simulink model "Ensamble_robot"  (R2016b)
settings: Solver=ode45  StartTime=0.0  StopTime=inf  RelTol=1e-3  EnableMultiTasking=on
undefined symbols (not defined in the file or in its folder): Brazo_1, Brazo_2, Ensamble_robot, Pinza, Pinza_1, RootPart, sigbuilder_block, Soporte, Torre
libraries: mblibv1 x28, simulink x12
settings Model: Creator=Alex3  LastModifiedBy=juan
settings DataIOCC: LimitDataPoints=on  SaveFormat=Array
settings OptimizationCC: LifeSpan=inf
settings DebuggingCC: SFUnexpectedBacktrackingDiag=warning  SFNoUnconditionalDefaultTransitionDiag=warning  SFExecutionAtInitializationDiag=none
settings HardwareCC: ProdBitPerPointer=32  ProdBitPerSizeT=32  ProdBitPerPtrDiffT=32  ProdLargestAtomicFloat=None  ProdIntDivRoundTo=Undefined  ProdEndianess=Unspecified  ProdWordSize=32  ProdHWDeviceType=32-bit Generic
settings ModelReferenceCC: PropagateSignalLabelsOutOfModel=off
settings GRTTargetCC: TargetLangStandard=C89/C90 (ANSI)  GeneratePreprocessorConditionals=Disable all
settings ConfigComp: CovMetricSettings=dw  CovHtmlReporting=on  CovSaveCumulativeToWorkspaceVar=on  CovSaveSingleToWorkspaceVar=on  CovExternalEMLEnable=off
settings SimMechanicsCC: VisOnUpdateDiagram=on  VisDuringSimulation=on
settings ConfigurationSet: Description=SimMechanics 2G

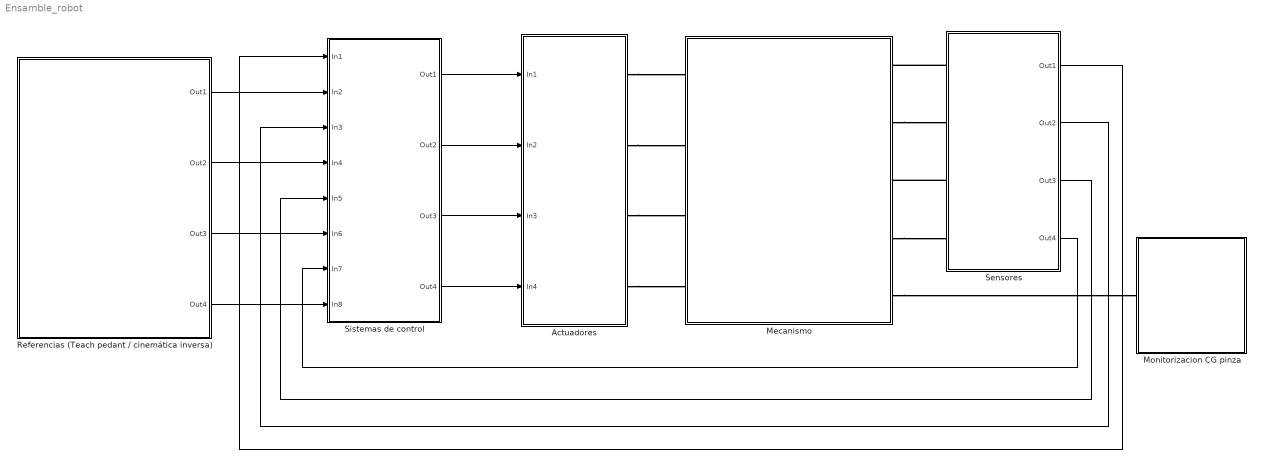
== system Ensamble_robot ==
  Actuadores : Subsystem
      mask Display: image('masks/motor.jpg');
  Mecanismo : Subsystem
      mask Display: image('masks/mascara_robot.png');
  "Monitorizacion CG pinza " : Subsystem
      mask Display: image('masks/orion_console_2_sm.jpg');
  Referencias (Teach pedant / cinemática inversa) : Subsystem
      mask Display: image('masks/_TEACHPD.GIF');
  Sensores : Subsystem
      mask Display: image('masks/encoders4.png');
  Sistemas de control : Subsystem
      mask Display: image('masks/pids4.png');
  wires:
  Sensores/1(Out1) -> Sistemas de control/1(In1)
  Sensores/2(Out2) -> Sistemas de control/3(In3)
  Sensores/3(Out3) -> Sistemas de control/5(In5)
  Sensores/4(Out4) -> Sistemas de control/7(In7)
  Sistemas de control/1(Out1) -> Actuadores/1(In1)
  Sistemas de control/2(Out2) -> Actuadores/2(In2)
  Sistemas de control/3(Out3) -> Actuadores/3(In3)
  Sistemas de control/4(Out4) -> Actuadores/4(In4)
  Referencias (Teach pedant / cinemática inversa)/1(Out1) -> Sistemas de control/2(In2)
  Referencias (Teach pedant / cinemática inversa)/2(Out2) -> Sistemas de control/4(In4)
  Referencias (Teach pedant / cinemática inversa)/3(Out3) -> Sistemas de control/6(In6)
  Referencias (Teach pedant / cinemática inversa)/4(Out4) -> Sistemas de control/8(In8)
  connections:
  Mecanismo/RConn5 -- "Monitorizacion CG pinza "/LConn1
  Actuadores/RConn1 -- Mecanismo/LConn1
  Actuadores/RConn2 -- Mecanismo/LConn2
  Actuadores/RConn3 -- Mecanismo/LConn3
  Actuadores/RConn4 -- Mecanismo/LConn4
  Sensores/LConn1 -- Mecanismo/RConn1
  Mecanismo/RConn2 -- Sensores/LConn2
  Sensores/LConn3 -- Mecanismo/RConn3
  Mecanismo/RConn4 -- Sensores/LConn4

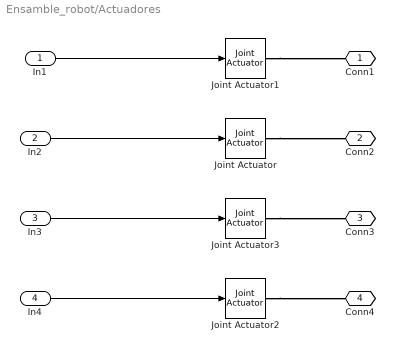
== system Ensamble_robot/Actuadores ==
  In1 : Inport
  In2 : Inport  Port=2
  In3 : Inport  Port=3
  In4 : Inport  Port=4
  Joint Actuator : mblibv1/Sensors &  Actuators/Joint Actuator  UpdateFromCAD=off  PhysicalDomain=Mechanical  PortType=blob  ActuationStyle=Motion  AngleUnits=deg  ArcVelocityUnits=deg/s  ArcAccelerationUnits=deg/s^2  CoordPositionUnits=mm  VelocityUnits=mm/s  AccelerationUnits=mm/s^2  ForceUnits=N  TorqueUnits=N*m  ActiveIO=on  Width=3  DialogClass=MechanicalActuatorBlock  Primitive=P1  ReferenceFrame=Absolute (World)
  Joint Actuator1 : mblibv1/Sensors &  Actuators/Joint Actuator  UpdateFromCAD=off  PhysicalDomain=Mechanical  PortType=blob  ActuationStyle=Motion  AngleUnits=rad  ArcVelocityUnits=rad/s  ArcAccelerationUnits=rad/s^2  CoordPositionUnits=mm  VelocityUnits=mm/s  AccelerationUnits=mm/s^2  ForceUnits=N  TorqueUnits=N*m  ActiveIO=on  Width=3  DialogClass=MechanicalActuatorBlock  Primitive=R1  ReferenceFrame=Absolute (World)
  Joint Actuator2 : mblibv1/Sensors &  Actuators/Joint Actuator  UpdateFromCAD=off  PhysicalDomain=Mechanical  PortType=blob  ActuationStyle=Motion  AngleUnits=rad  ArcVelocityUnits=rad/s  ArcAccelerationUnits=rad/s^2  CoordPositionUnits=mm  VelocityUnits=mm/s  AccelerationUnits=mm/s^2  ForceUnits=N  TorqueUnits=N*m  ActiveIO=on  Width=3  DialogClass=MechanicalActuatorBlock  Primitive=R1  ReferenceFrame=Absolute (World)
  Joint Actuator3 : mblibv1/Sensors &  Actuators/Joint Actuator  UpdateFromCAD=off  PhysicalDomain=Mechanical  PortType=blob  ActuationStyle=Motion  AngleUnits=rad  ArcVelocityUnits=rad/s  ArcAccelerationUnits=rad/s^2  CoordPositionUnits=mm  VelocityUnits=mm/s  AccelerationUnits=mm/s^2  ForceUnits=N  TorqueUnits=N*m  ActiveIO=on  Width=3  DialogClass=MechanicalActuatorBlock  Primitive=R1  ReferenceFrame=Absolute (World)
  Conn1 : PMIOPort  Port=1  Side=Right
  Conn2 : PMIOPort  Port=2  Side=Right
  Conn3 : PMIOPort  Port=3  Side=Right
  Conn4 : PMIOPort  Port=4  Side=Right
  wires:
  In1/1 -> Joint Actuator1/1
  In4/1 -> Joint Actuator2/1
  In3/1 -> Joint Actuator3/1
  In2/1 -> Joint Actuator/1
  connections:
  Joint Actuator2/RConn1 -- Conn4/RConn1
  Joint Actuator1/RConn1 -- Conn1/RConn1
  Joint Actuator3/RConn1 -- Conn3/RConn1
  Joint Actuator/RConn1 -- Conn2/RConn1

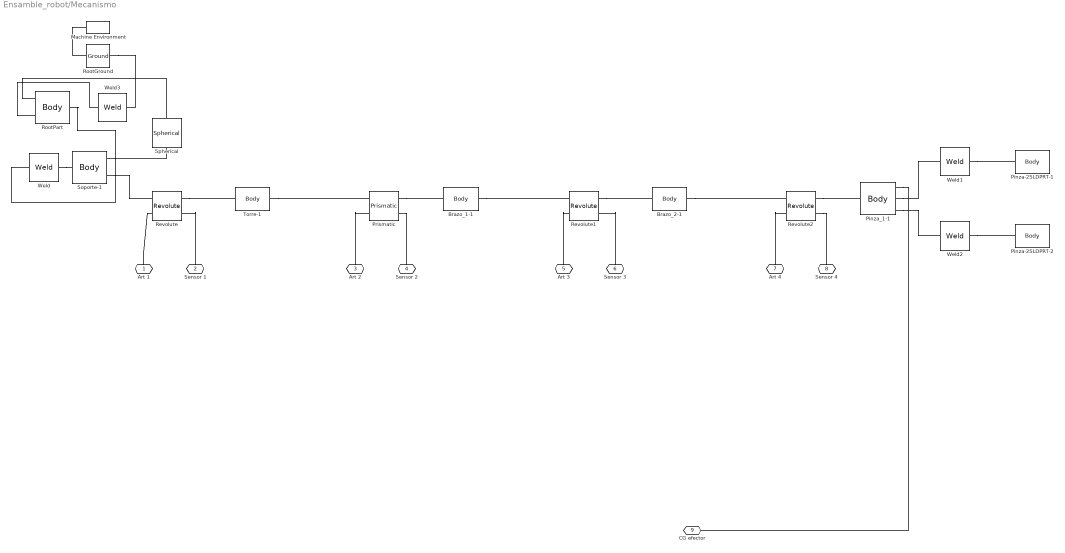
== system Ensamble_robot/Mecanismo ==
  Brazo_1-1 : mblibv1/Bodies/Body  LConnTagsString=CS2  RConnTagsString=CS3  UpdateFromCAD=on  PMImportedID=Brazo_1-1  DialogClass=MechanicalBodyBlock  Mass=5.04274  MassUnits=kg  InertiaUnits=kg*m^2  Inertia=[0.0173518,0.0122763,1.33704e-09;0.0122763,0.106444,-1.19326e-09;1.33704e-09,-1.19326e-09,0.102671]  Shape=Cylinder  ShapeDims=[1 1]  ShapeUnits=m  ShapeUse=false  Density=1  DensityUnits=kg/m^3  DensityUse=false  GraphicsMode=GFXFILE  GraphicsFileName=Ensamble_robot - Brazo_1-1.STL  BodyColorSelMode=COLORPALETTE  BodyColor=[1;1;1]  AttachedToCS=CS1  CG=Right$CG$[0.204832 0.0464629 2.69197e-09]$WORLD$WORLD$m$[1 0 0;0 1 0;0 0 1]$3x3 Transform$rad$WORLD$false$Brazo_1-1::CG(AUTOGEN)  WorkingFrames=Right$CS1$[0.45 0.0499751 0]$WORLD$WORLD$m$[1 0 0;0 1 0;0 0 1]$3x3 Transform$rad$WORLD$false$Brazo_1-1::CS1(AUTOGEN)#Left$CS2$[0 0.149975 0.045]$WORLD$WORLD$m$[1 0 0;0 1 0;0 0 1]$3x3 Transform$rad$WORLD$true$Brazo_1-1:-:Torre-1::Brazo_1-1(AUTOGEN)#Right$CS3$[0.45 0.0299751 0]$WORLD$WORLD$m$[1 0 0;0 1 0;0 0 1]$3x3 Transform$rad$WORLD$true$Brazo_1-1:-:Brazo_2-1::Brazo_1-1(AUTOGEN)  CGPos=[0.204832 0.0464629 2.69197e-09]  CGRot=[1 0 0;0 1 0;0 0 1]  CS0Pos=[]  CS0Rot=[]  CS1Pos=[0.45 0.0499751 0]  CS1Rot=[1 0 0;0 1 0;0 0 1]  CS2Pos=[0 0.149975 0.045]  CS2Rot=[1 0 0;0 1 0;0 0 1]  CS3Pos=[0.45 0.0299751 0]  CS3Rot=[1 0 0;0 1 0;0 0 1]  CS4Pos=[]  CS4Rot=[]  CS5Pos=[]  CS5Rot=[]  CS6Pos=[]  CS6Rot=[]  CS7Pos=[]  CS7Rot=[]  CS8Pos=[]  CS8Rot=[]  CS9Pos=[]  CS9Rot=[]  CS10Pos=[]  CS10Rot=[]  CS11Pos=[]  CS11Rot=[]  CS12Pos=[]  CS12Rot=[]  CS13Pos=[]  CS13Rot=[]  CS14Pos=[]  CS14Rot=[]  CS15Pos=[]  CS15Rot=[]  CS16Pos=[]  CS16Rot=[]  CS17Pos=[]  CS17Rot=[]  CS18Pos=[]  CS18Rot=[]  CS19Pos=[]  CS19Rot=[]  CS20Pos=[]  CS20Rot=[]
  Brazo_2-1 : mblibv1/Bodies/Body  LConnTagsString=CS2  RConnTagsString=CS3  UpdateFromCAD=on  PMImportedID=Brazo_2-1  DialogClass=MechanicalBodyBlock  Mass=1.88667  MassUnits=kg  InertiaUnits=kg*m^2  Inertia=[0.00269492,0.000426403,-1.18231e-09;0.000426403,0.0126019,2.20098e-09;-1.18231e-09,2.20098e-09,0.0117797]  Shape=Cylinder  ShapeDims=[1 1]  ShapeUnits=m  ShapeUse=false  Density=1  DensityUnits=kg/m^3  DensityUse=false  GraphicsMode=GFXFILE  GraphicsFileName=Ensamble_robot - Brazo_2-1.STL  BodyColorSelMode=COLORPALETTE  BodyColor=[1;1;1]  AttachedToCS=CS1  CG=Right$CG$[0.507024 -0.0192513 -1.13579e-08]$WORLD$WORLD$m$[1 0 0;0 1 0;0 0 1]$3x3 Transform$rad$WORLD$false$Brazo_2-1::CG(AUTOGEN)  WorkingFrames=Right$CS1$[0.45 -0.0500249 0]$WORLD$WORLD$m$[1 0 0;0 1 0;0 0 1]$3x3 Transform$rad$WORLD$false$Brazo_2-1::CS1(AUTOGEN)#Left$CS2$[0.45 0.0299751 0]$WORLD$WORLD$m$[1 0 0;0 1 0;0 0 1]$3x3 Transform$rad$WORLD$true$Brazo_1-1:-:Brazo_2-1::Brazo_2-1(AUTOGEN)#Right$CS3$[0.65 -0.0200249 0]$WORLD$WORLD$m$[1 0 0;0 1 0;0 0 1]$3x3 Transform$rad$WORLD$true$Brazo_2-1:-:Pinza_1-1::Brazo_2-1(AUTOGEN)  CGPos=[0.507024 -0.0192513 -1.13579e-08]  CGRot=[1 0 0;0 1 0;0 0 1]  CS0Pos=[]  CS0Rot=[]  CS1Pos=[0.45 -0.0500249 0]  CS1Rot=[1 0 0;0 1 0;0 0 1]  CS2Pos=[0.45 0.0299751 0]  CS2Rot=[1 0 0;0 1 0;0 0 1]  CS3Pos=[0.65 -0.0200249 0]  CS3Rot=[1 0 0;0 1 0;0 0 1]  CS4Pos=[]  CS4Rot=[]  CS5Pos=[]  CS5Rot=[]  CS6Pos=[]  CS6Rot=[]  CS7Pos=[]  CS7Rot=[]  CS8Pos=[]  CS8Rot=[]  CS9Pos=[]  CS9Rot=[]  CS10Pos=[]  CS10Rot=[]  CS11Pos=[]  CS11Rot=[]  CS12Pos=[]  CS12Rot=[]  CS13Pos=[]  CS13Rot=[]  CS14Pos=[]  CS14Rot=[]  CS15Pos=[]  CS15Rot=[]  CS16Pos=[]  CS16Rot=[]  CS17Pos=[]  CS17Rot=[]  CS18Pos=[]  CS18Rot=[]  CS19Pos=[]  CS19Rot=[]  CS20Pos=[]  CS20Rot=[]
  Machine Environment : mblibv1/Bodies/Machine Environment  PortType=env  PhysicalDomain=Mechanical  DialogTemplateClass=MECH.MachineEnvironment  SyncWhenCopied=off  Gravity=[0 -9.81 0]  GravityUnits=m/s^2  GravityAsSignal=off  Dimensionality=Auto-detect  AnalysisType=Forward dynamics  LinearAssemblyTolerance=1e-3  LinearAssemblyToleranceUnits=m  AngularAssemblyTolerance=1e-3  AngularAssemblyToleranceUnits=rad  ConstraintSolverType=Stabilizing  ConstraintRelTolerance=1e-4  ConstraintAbsTolerance=1e-4  UseRobustSingularityHandling=off  RedundancyAnalysisToleranceType=Automatically select tolerance  RedundancyAnalysisTolerance=1e-14  StatePerturbationType=Fixed  PerturbationSize=1e-5  VisualizeMachine=on  BodyVisualizationType=Use model default body geometries  BodyColorSelMode=Use model default  DefaultBodyColor=[1 0 0]
  Pinza-2SLDPRT-1 : mblibv1/Bodies/Body  LConnTagsString=CS2  UpdateFromCAD=on  PMImportedID=Pinza-2SLDPRT-1  DialogClass=MechanicalBodyBlock  Mass=0.01755  MassUnits=kg  InertiaUnits=kg*m^2  Inertia=[5.56763e-07,0,0;0,7.2684e-06,0;0,0,6.78476e-06]  Shape=Cylinder  ShapeDims=[1 1]  ShapeUnits=m  ShapeUse=false  Density=1  DensityUnits=kg/m^3  DensityUse=false  GraphicsMode=GFXFILE  GraphicsFileName=Ensamble_robot - Pinza-2SLDPRT-1.STL  BodyColorSelMode=COLORPALETTE  BodyColor=[0.894118;0.913725;0.929412]  AttachedToCS=CS1  CG=Right$CG$[0.705013 -0.0950249 -0.0525]$WORLD$WORLD$m$[1 0 0;0 0 1;0 -1 0]$3x3 Transform$rad$WORLD$false$Pinza-2SLDPRT-1::CG(AUTOGEN)  WorkingFrames=Right$CS1$[0.697 -0.0950249 -0.05]$WORLD$WORLD$m$[1 0 0;0 0 1;0 -1 0]$3x3 Transform$rad$WORLD$false$Pinza-2SLDPRT-1::CS1(AUTOGEN)#Left$CS2$[0.672 -0.105025 -0.055]$WORLD$WORLD$m$[1 0 0;0 1 0;0 0 1]$3x3 Transform$rad$WORLD$true$Pinza-2SLDPRT-1:-:Pinza_1-1::Pinza-2SLDPRT-1(AUTOGEN)  CGPos=[0.705013 -0.0950249 -0.0525]  CGRot=[1 0 0;0 0 1;0 -1 0]  CS0Pos=[]  CS0Rot=[]  CS1Pos=[0.697 -0.0950249 -0.05]  CS1Rot=[1 0 0;0 0 1;0 -1 0]  CS2Pos=[0.672 -0.105025 -0.055]  CS2Rot=[1 0 0;0 1 0;0 0 1]  CS3Pos=[]  CS3Rot=[]  CS4Pos=[]  CS4Rot=[]  CS5Pos=[]  CS5Rot=[]  CS6Pos=[]  CS6Rot=[]  CS7Pos=[]  CS7Rot=[]  CS8Pos=[]  CS8Rot=[]  CS9Pos=[]  CS9Rot=[]  CS10Pos=[]  CS10Rot=[]  CS11Pos=[]  CS11Rot=[]  CS12Pos=[]  CS12Rot=[]  CS13Pos=[]  CS13Rot=[]  CS14Pos=[]  CS14Rot=[]  CS15Pos=[]  CS15Rot=[]  CS16Pos=[]  CS16Rot=[]  CS17Pos=[]  CS17Rot=[]  CS18Pos=[]  CS18Rot=[]  CS19Pos=[]  CS19Rot=[]  CS20Pos=[]  CS20Rot=[]
  Pinza-2SLDPRT-2 : mblibv1/Bodies/Body  LConnTagsString=CS2  UpdateFromCAD=on  PMImportedID=Pinza-2SLDPRT-2  DialogClass=MechanicalBodyBlock  Mass=0.01755  MassUnits=kg  InertiaUnits=kg*m^2  Inertia=[5.56763e-07,0,0;0,7.2684e-06,0;0,0,6.78476e-06]  Shape=Cylinder  ShapeDims=[1 1]  ShapeUnits=m  ShapeUse=false  Density=1  DensityUnits=kg/m^3  DensityUse=false  GraphicsMode=GFXFILE  GraphicsFileName=Ensamble_robot - Pinza-2SLDPRT-2.STL  BodyColorSelMode=COLORPALETTE  BodyColor=[0.894118;0.913725;0.929412]  AttachedToCS=CS1  CG=Right$CG$[0.705013 -0.0950249 0.0525]$WORLD$WORLD$m$[1 0 0;0 0 -1;0 1 0]$3x3 Transform$rad$WORLD$false$Pinza-2SLDPRT-2::CG(AUTOGEN)  WorkingFrames=Right$CS1$[0.697 -0.0950249 0.05]$WORLD$WORLD$m$[1 0 0;0 0 -1;0 1 0]$3x3 Transform$rad$WORLD$false$Pinza-2SLDPRT-2::CS1(AUTOGEN)#Left$CS2$[0.672 -0.105025 0.055]$WORLD$WORLD$m$[1 0 0;0 1 0;0 0 1]$3x3 Transform$rad$WORLD$true$Pinza-2SLDPRT-2:-:Pinza_1-1::Pinza-2SLDPRT-2(AUTOGEN)  CGPos=[0.705013 -0.0950249 0.0525]  CGRot=[1 0 0;0 0 -1;0 1 0]  CS0Pos=[]  CS0Rot=[]  CS1Pos=[0.697 -0.0950249 0.05]  CS1Rot=[1 0 0;0 0 -1;0 1 0]  CS2Pos=[0.672 -0.105025 0.055]  CS2Rot=[1 0 0;0 1 0;0 0 1]  CS3Pos=[]  CS3Rot=[]  CS4Pos=[]  CS4Rot=[]  CS5Pos=[]  CS5Rot=[]  CS6Pos=[]  CS6Rot=[]  CS7Pos=[]  CS7Rot=[]  CS8Pos=[]  CS8Rot=[]  CS9Pos=[]  CS9Rot=[]  CS10Pos=[]  CS10Rot=[]  CS11Pos=[]  CS11Rot=[]  CS12Pos=[]  CS12Rot=[]  CS13Pos=[]  CS13Rot=[]  CS14Pos=[]  CS14Rot=[]  CS15Pos=[]  CS15Rot=[]  CS16Pos=[]  CS16Rot=[]  CS17Pos=[]  CS17Rot=[]  CS18Pos=[]  CS18Rot=[]  CS19Pos=[]  CS19Rot=[]  CS20Pos=[]  CS20Rot=[]
  Pinza_1-1 : mblibv1/Bodies/Body  LConnTagsString=CS2  RConnTagsString=CG|CS3|CS4  UpdateFromCAD=on  PMImportedID=Pinza_1-1  DialogClass=MechanicalBodyBlock  Mass=1.1552  MassUnits=kg  InertiaUnits=kg*m^2  Inertia=[0.00139548,9.82419e-05,0;9.82419e-05,0.00107204,0;0,0,0.00130274]  Shape=Cylinder  ShapeDims=[1 1]  ShapeUnits=m  ShapeUse=false  Density=1  DensityUnits=kg/m^3  DensityUse=false  GraphicsMode=GFXFILE  GraphicsFileName=Ensamble_robot - Pinza_1-1.STL  BodyColorSelMode=COLORPALETTE  BodyColor=[0.89412 0.91373 0.92941]  AttachedToCS=CS1  CG=Right$CG$[0.653502 -0.0707388 0]$WORLD$WORLD$m$[1 0 0;0 1 0;0 0 1]$3x3 Transform$rad$WORLD$true$Pinza_1-1::CG(AUTOGEN)  WorkingFrames=Right$CS1$[0.65 -0.110025 0]$WORLD$WORLD$m$[1 0 0;0 1 0;0 0 1]$3x3 Transform$rad$WORLD$false$Pinza_1-1::CS1(AUTOGEN)#Left$CS2$[0.65 -0.0200249 0]$WORLD$WORLD$m$[1 0 0;0 1 0;0 0 1]$3x3 Transform$rad$WORLD$true$Brazo_2-1:-:Pinza_1-1::Pinza_1-1(AUTOGEN)#Right$CS3$[0.672 -0.105025 -0.055]$WORLD$WORLD$m$[1 0 0;0 1 0;0 0 1]$3x3 Transform$rad$WORLD$true$Pinza-2SLDPRT-1:-:Pinza_1-1::Pinza_1-1(AUTOGEN)#Right$CS4$[0.672 -0.105025 0.055]$WORLD$WORLD$m$[1 0 0;0 1 0;0 0 1]$3x3 Transform$rad$WORLD$true$Pinza-2SLDPRT-2:-:Pinza_1-1::Pinza_1-1(AUTOGEN)  CGPos=[0.653502 -0.0707388 0]  CGRot=[1 0 0;0 1 0;0 0 1]  CS0Pos=[]  CS0Rot=[]  CS1Pos=[0.65 -0.110025 0]  CS1Rot=[1 0 0;0 1 0;0 0 1]  CS2Pos=[0.65 -0.0200249 0]  CS2Rot=[1 0 0;0 1 0;0 0 1]  CS3Pos=[0.672 -0.105025 -0.055]  CS3Rot=[1 0 0;0 1 0;0 0 1]  CS4Pos=[0.672 -0.105025 0.055]  CS4Rot=[1 0 0;0 1 0;0 0 1]  CS5Pos=[]  CS5Rot=[]  CS6Pos=[]  CS6Rot=[]  CS7Pos=[]  CS7Rot=[]  CS8Pos=[]  CS8Rot=[]  CS9Pos=[]  CS9Rot=[]  CS10Pos=[]  CS10Rot=[]  CS11Pos=[]  CS11Rot=[]  CS12Pos=[]  CS12Rot=[]  CS13Pos=[]  CS13Rot=[]  CS14Pos=[]  CS14Rot=[]  CS15Pos=[]  CS15Rot=[]  CS16Pos=[]  CS16Rot=[]  CS17Pos=[]  CS17Rot=[]  CS18Pos=[]  CS18Rot=[]  CS19Pos=[]  CS19Rot=[]  CS20Pos=[]  CS20Rot=[]
  Prismatic : mblibv1/Joints/Prismatic  LConnTagsString=__newl0|SA1  RConnTagsString=__newr0|SA1  UpdateFromCAD=on  PMImportedID=Brazo_1-1:-:Torre-1  NumSAPorts=2  CutJoint=off  MarkAsCut=off  Primitives=prismatic  PrimitiveProps=P1$World$[0,-1,0]$prismatic  DialogClass=JointBlock  P1Axis=[0,-1,0]
  Revolute : mblibv1/Joints/Revolute  LConnTagsString=__newl0|SA1  RConnTagsString=__newr0|SA1  UpdateFromCAD=on  PMImportedID=Soporte-1:-:Torre-1  NumSAPorts=2  CutJoint=off  MarkAsCut=off  Primitives=prismatic  PrimitiveProps=R1$World$[0,-1,0]$revolute  DialogClass=JointBlock  R1Axis=[0,-1,0]
  Revolute1 : mblibv1/Joints/Revolute  LConnTagsString=__newl0|SA1  RConnTagsString=__newr0|SA1  UpdateFromCAD=on  PMImportedID=Brazo_1-1:-:Brazo_2-1  NumSAPorts=2  CutJoint=off  MarkAsCut=off  Primitives=prismatic  PrimitiveProps=R1$World$[0,-1,0]$revolute  DialogClass=JointBlock  R1Axis=[0,-1,0]
  Revolute2 : mblibv1/Joints/Revolute  LConnTagsString=__newl0|SA1  RConnTagsString=__newr0|SA1  UpdateFromCAD=on  PMImportedID=Brazo_2-1:-:Pinza_1-1  NumSAPorts=2  CutJoint=off  MarkAsCut=off  Primitives=prismatic  PrimitiveProps=R1$World$[0,-1,0]$revolute  DialogClass=JointBlock  R1Axis=[0,-1,0]
  RootGround : mblibv1/Bodies/Ground  UpdateFromCAD=on  PMImportedID=RootGround  LeftPortType=env  RightPortType=workingframe  PhysicalDomain=Mechanical  DialogClass=GroundBlock  CoordPosition=[0.0659419,0.00229338,1.11665e-06]  CoordPositionUnits=m  StateVectorMgrId=-1  MachineId=[0 0]  ShowEnvPort=on  ParameterChecksum=[1902267943, 726416014, 765096310, 2272254341]  TopologyChecksum=[1063915244, 2503524642, 3963338569, 4138555748]
  RootPart : mblibv1/Bodies/Body  LConnTagsString=CS3|CS4  RConnTagsString=CS2  UpdateFromCAD=on  PMImportedID=Ensamble_robot/RootPart  DialogClass=MechanicalBodyBlock  Mass=0  MassUnits=kg  InertiaUnits=kg*m^2  Inertia=[0,0,0;0,0,0;0,0,0]  Shape=Cylinder  ShapeDims=[1 1]  ShapeUnits=m  ShapeUse=false  Density=1  DensityUnits=kg/m^3  DensityUse=false  GraphicsMode=MACHINE_DEFAULT  BodyColorSelMode=MACHINE_DEFAULT  BodyColor=[1;0;0]  AttachedToCS=CS1  CG=Right$CG$[0.0659419 0.00229338 1.11665e-06]$WORLD$WORLD$m$[1 0 0;0 1 0;0 0 1]$3x3 Transform$rad$WORLD$false$Ensamble_robot/RootPart::CG(AUTOGEN)  WorkingFrames=Right$CS1$[0 0 0]$WORLD$WORLD$m$[1 0 0;0 1 0;0 0 1]$3x3 Transform$rad$WORLD$false$Ensamble_robot/RootPart::CS1(AUTOGEN)#Right$CS2$[-0.119346 -0.242891 4.53911e-06]$WORLD$WORLD$m$[1 0 0;0 1 0;0 0 1]$3x3 Transform$rad$WORLD$true$Ensamble_robot/RootPart:-:Soporte-1::Ensamble_robot/RootPart(AUTOGEN)#Left$CS3$[0 0 0]$WORLD$WORLD$m$[1 0 0;0 1 0;0 0 1]$3x3 Transform$rad$WORLD$true$:-:Ensamble_robot/RootPart::Ensamble_robot/RootPart(AUTOGEN)#Left$CS4$[0.0659419 0.00229338 1.11665e-06]$WORLD$WORLD$m$[1 0 0;0 1 0;0 0 1]$3x3 Transform$rad$WORLD$true$Ensamble_robot/RootPart:-:RootGround::Ensamble_robot/RootPart(AUTOGEN)  CGPos=[0.0659419 0.00229338 1.11665e-06]  CGRot=[1 0 0;0 1 0;0 0 1]  CS0Pos=[]  CS0Rot=[]  CS1Pos=[0 0 0]  CS1Rot=[1 0 0;0 1 0;0 0 1]  CS2Pos=[-0.119346 -0.242891 4.53911e-06]  CS2Rot=[1 0 0;0 1 0;0 0 1]  CS3Pos=[0 0 0]  CS3Rot=[1 0 0;0 1 0;0 0 1]  CS4Pos=[0.0659419 0.00229338 1.11665e-06]  CS4Rot=[1 0 0;0 1 0;0 0 1]  CS5Pos=[]  CS5Rot=[]  CS6Pos=[]  CS6Rot=[]  CS7Pos=[]  CS7Rot=[]  CS8Pos=[]  CS8Rot=[]  CS9Pos=[]  CS9Rot=[]  CS10Pos=[]  CS10Rot=[]  CS11Pos=[]  CS11Rot=[]  CS12Pos=[]  CS12Rot=[]  CS13Pos=[]  CS13Rot=[]  CS14Pos=[]  CS14Rot=[]  CS15Pos=[]  CS15Rot=[]  CS16Pos=[]  CS16Rot=[]  CS17Pos=[]  CS17Rot=[]  CS18Pos=[]  CS18Rot=[]  CS19Pos=[]  CS19Rot=[]  CS20Pos=[]  CS20Rot=[]
  Soporte-1 : mblibv1/Bodies/Body  LConnTagsString=CS2  RConnTagsString=CS3|CS4  UpdateFromCAD=on  PMImportedID=Soporte-1  DialogClass=MechanicalBodyBlock  Mass=6.83887  MassUnits=kg  InertiaUnits=kg*m^2  Inertia=[0.0271292,0.00214532,-1.0763e-06;0.00214532,0.102791,-1.48243e-06;-1.0763e-06,-1.48243e-06,0.0878129]  Shape=Cylinder  ShapeDims=[1 1]  ShapeUnits=m  ShapeUse=false  Density=1  DensityUnits=kg/m^3  DensityUse=false  GraphicsMode=GFXFILE  GraphicsFileName=Ensamble_robot - Soporte-1.STL  BodyColorSelMode=COLORPALETTE  BodyColor=[1;1;1]  AttachedToCS=CS1  CG=Right$CG$[-0.119346 -0.242891 4.53911e-06]$WORLD$WORLD$m$[1 0 0;0 1 0;0 0 1]$3x3 Transform$rad$WORLD$false$Soporte-1::CG(AUTOGEN)  WorkingFrames=Right$CS1$[0 -0.29 0]$WORLD$WORLD$m$[1 0 0;0 1 0;0 0 1]$3x3 Transform$rad$WORLD$false$Soporte-1::CS1(AUTOGEN)#Left$CS2$[-0.119346 -0.242891 4.53911e-06]$WORLD$WORLD$m$[1 0 0;0 1 0;0 0 1]$3x3 Transform$rad$WORLD$true$Ensamble_robot/RootPart:-:Soporte-1::Soporte-1(AUTOGEN)#Right$CS3$[0 0 0]$WORLD$WORLD$m$[1 0 0;0 1 0;0 0 1]$3x3 Transform$rad$WORLD$true$:-:Ensamble_robot/RootPart::Soporte-1(AUTOGEN)#Right$CS4$[0 -0.23 0]$WORLD$WORLD$m$[1 0 0;0 1 0;0 0 1]$3x3 Transform$rad$WORLD$true$Soporte-1:-:Torre-1::Soporte-1(AUTOGEN)  CGPos=[-0.119346 -0.242891 4.53911e-06]  CGRot=[1 0 0;0 1 0;0 0 1]  CS0Pos=[]  CS0Rot=[]  CS1Pos=[0 -0.29 0]  CS1Rot=[1 0 0;0 1 0;0 0 1]  CS2Pos=[-0.119346 -0.242891 4.53911e-06]  CS2Rot=[1 0 0;0 1 0;0 0 1]  CS3Pos=[0 0 0]  CS3Rot=[1 0 0;0 1 0;0 0 1]  CS4Pos=[0 -0.23 0]  CS4Rot=[1 0 0;0 1 0;0 0 1]  CS5Pos=[]  CS5Rot=[]  CS6Pos=[]  CS6Rot=[]  CS7Pos=[]  CS7Rot=[]  CS8Pos=[]  CS8Rot=[]  CS9Pos=[]  CS9Rot=[]  CS10Pos=[]  CS10Rot=[]  CS11Pos=[]  CS11Rot=[]  CS12Pos=[]  CS12Rot=[]  CS13Pos=[]  CS13Rot=[]  CS14Pos=[]  CS14Rot=[]  CS15Pos=[]  CS15Rot=[]  CS16Pos=[]  CS16Rot=[]  CS17Pos=[]  CS17Rot=[]  CS18Pos=[]  CS18Rot=[]  CS19Pos=[]  CS19Rot=[]  CS20Pos=[]  CS20Rot=[]
  Spherical : mblibv1/Joints/Spherical  LConnTagsString=__newl0  RConnTagsString=__newr0  UpdateFromCAD=on  PMImportedID=:-:Ensamble_robot/RootPart  NumSAPorts=0  CutJoint=off  MarkAsCut=off  Primitives=spherical  PrimitiveProps=S$WORLD$[0,0,0]$spherical  DialogClass=JointBlock  SAxis=[0,0,0]
  Torre-1 : mblibv1/Bodies/Body  LConnTagsString=CS2  RConnTagsString=CS3  UpdateFromCAD=on  PMImportedID=Torre-1  DialogClass=MechanicalBodyBlock  Mass=12.906  MassUnits=kg  InertiaUnits=kg*m^2  Inertia=[0.653453,0.0144429,-5.6767e-09;0.0144429,0.0391342,-1.12795e-08;-5.6767e-09,-1.12795e-08,0.64837]  Shape=Cylinder  ShapeDims=[1 1]  ShapeUnits=m  ShapeUse=false  Density=1  DensityUnits=kg/m^3  DensityUse=false  GraphicsMode=GFXFILE  GraphicsFileName=Ensamble_robot - Torre-1.STL  BodyColorSelMode=COLORPALETTE  BodyColor=[1;1;1]  AttachedToCS=CS1  CG=Right$CG$[-0.00895228 0.124909 6.2308e-09]$WORLD$WORLD$m$[1 0 0;0 1 0;0 0 1]$3x3 Transform$rad$WORLD$false$Torre-1::CG(AUTOGEN)  WorkingFrames=Right$CS1$[0 -0.18 0]$WORLD$WORLD$m$[1 0 0;0 1 0;0 0 1]$3x3 Transform$rad$WORLD$false$Torre-1::CS1(AUTOGEN)#Left$CS2$[0 -0.23 0]$WORLD$WORLD$m$[1 0 0;0 1 0;0 0 1]$3x3 Transform$rad$WORLD$true$Soporte-1:-:Torre-1::Torre-1(AUTOGEN)#Right$CS3$[0 0.5 0.045]$WORLD$WORLD$m$[1 0 0;0 1 0;0 0 1]$3x3 Transform$rad$WORLD$true$Brazo_1-1:-:Torre-1::Torre-1(AUTOGEN)  CGPos=[-0.00895228 0.124909 6.2308e-09]  CGRot=[1 0 0;0 1 0;0 0 1]  CS0Pos=[]  CS0Rot=[]  CS1Pos=[0 -0.18 0]  CS1Rot=[1 0 0;0 1 0;0 0 1]  CS2Pos=[0 -0.23 0]  CS2Rot=[1 0 0;0 1 0;0 0 1]  CS3Pos=[0 0.5 0.045]  CS3Rot=[1 0 0;0 1 0;0 0 1]  CS4Pos=[]  CS4Rot=[]  CS5Pos=[]  CS5Rot=[]  CS6Pos=[]  CS6Rot=[]  CS7Pos=[]  CS7Rot=[]  CS8Pos=[]  CS8Rot=[]  CS9Pos=[]  CS9Rot=[]  CS10Pos=[]  CS10Rot=[]  CS11Pos=[]  CS11Rot=[]  CS12Pos=[]  CS12Rot=[]  CS13Pos=[]  CS13Rot=[]  CS14Pos=[]  CS14Rot=[]  CS15Pos=[]  CS15Rot=[]  CS16Pos=[]  CS16Rot=[]  CS17Pos=[]  CS17Rot=[]  CS18Pos=[]  CS18Rot=[]  CS19Pos=[]  CS19Rot=[]  CS20Pos=[]  CS20Rot=[]
  Weld : mblibv1/Joints/Weld  LConnTagsString=__newl0  RConnTagsString=__newr0  UpdateFromCAD=on  PMImportedID=Ensamble_robot/RootPart:-:Soporte-1  NumSAPorts=0  CutJoint=off  MarkAsCut=off  Primitives=weld  PrimitiveProps=W$WORLD$[0.57735,0.57735,0.57735]$weld  DialogClass=JointBlock  WAxis=[0.57735,0.57735,0.57735]
  Weld1 : mblibv1/Joints/Weld  LConnTagsString=__newl0  RConnTagsString=__newr0  UpdateFromCAD=on  PMImportedID=Pinza-2SLDPRT-1:-:Pinza_1-1  NumSAPorts=0  CutJoint=off  MarkAsCut=off  Primitives=weld  PrimitiveProps=W$WORLD$[0.57735,0.57735,0.57735]$weld  DialogClass=JointBlock  WAxis=[0.57735,0.57735,0.57735]
  Weld2 : mblibv1/Joints/Weld  LConnTagsString=__newl0  RConnTagsString=__newr0  UpdateFromCAD=on  PMImportedID=Pinza-2SLDPRT-2:-:Pinza_1-1  NumSAPorts=0  CutJoint=off  MarkAsCut=off  Primitives=weld  PrimitiveProps=W$WORLD$[0.57735,0.57735,0.57735]$weld  DialogClass=JointBlock  WAxis=[0.57735,0.57735,0.57735]
  Weld3 : mblibv1/Joints/Weld  LConnTagsString=__newl0  RConnTagsString=__newr0  UpdateFromCAD=on  PMImportedID=Ensamble_robot/RootPart:-:RootGround  NumSAPorts=0  CutJoint=off  MarkAsCut=off  Primitives=weld  PrimitiveProps=W$WORLD$[0.57735,0.57735,0.57735]$weld  DialogClass=JointBlock  WAxis=[0.57735,0.57735,0.57735]
  Art 1 : PMIOPort  Port=1  Side=Left
  Sensor 1 : PMIOPort  Port=2  Side=Right
  Art 2 : PMIOPort  Port=3  Side=Left
  Sensor 2 : PMIOPort  Port=4  Side=Right
  Art 3 : PMIOPort  Port=5  Side=Left
  Sensor 3 : PMIOPort  Port=6  Side=Right
  Art 4 : PMIOPort  Port=7  Side=Left
  Sensor 4 : PMIOPort  Port=8  Side=Right
  CG efector : PMIOPort  Port=9  Side=Right
  connections:
  Soporte-1/RConn2 -- Revolute/LConn1
  Soporte-1/RConn1 -- Spherical/LConn1
  Sensor 3/RConn1 -- Revolute1/RConn2
  Revolute2/RConn2 -- Sensor 4/RConn1
  Weld2/RConn1 -- Pinza-2SLDPRT-2/LConn1
  Spherical/RConn1 -- RootPart/LConn1
  Revolute2/RConn1 -- Pinza_1-1/LConn1
  RootPart/RConn1 -- Weld/LConn1
  Prismatic/RConn2 -- Sensor 2/RConn1
  Torre-1/RConn1 -- Prismatic/LConn1
  Art 3/RConn1 -- Revolute1/LConn2
  Brazo_2-1/RConn1 -- Revolute2/LConn1
  Pinza_1-1/RConn3 -- Weld2/LConn1
  Weld1/RConn1 -- Pinza-2SLDPRT-1/LConn1
  RootGround/RConn1 -- Weld3/LConn1
  Art 4/RConn1 -- Revolute2/LConn2
  Revolute1/RConn1 -- Brazo_2-1/LConn1
  RootGround/LConn1 -- Machine Environment/RConn1
  Prismatic/RConn1 -- Brazo_1-1/LConn1
  Pinza_1-1/RConn1 -- CG efector/RConn1
  Art 2/RConn1 -- Prismatic/LConn2
  Weld/RConn1 -- Soporte-1/LConn1
  Weld3/RConn1 -- RootPart/LConn2
  Revolute/RConn1 -- Torre-1/LConn1
  Sensor 1/RConn1 -- Revolute/RConn2
  Pinza_1-1/RConn2 -- Weld1/LConn1
  Art 1/RConn1 -- Revolute/LConn2
  Brazo_1-1/RConn1 -- Revolute1/LConn1

== system Ensamble_robot/Monitorizacion CG pinza  ==
  Altura leída : Display
  Body Sensor : mblibv1/Sensors &  Actuators/Body Sensor  UpdateFromCAD=off  PhysicalDomain=Mechanical  PortType=blob  Muxed=on  Pose=off  Angle=on  AngleUnits=deg  ArcVelocity=off  ArcVelocityUnits=deg/s  ArcAcceleration=off  ArcAccelerationUnits=deg/s^2  CoordPosition=on  CoordPositionUnits=mm  Velocity=off  VelocityUnits=m/s  Acceleration=off  AccelerationUnits=m/s^2  Quaternion=on  QuaternionDT=off  QuaternionDDT=off  QuaternionUnits=off  OutputVector=[1]  ActiveIO=on  Width=3  DialogClass=MechanicalSensorBlock  ReferenceFrame=Absolute (World)
  Demux : Demux  Outputs=3
  Posición X leída : Display
  Posición Z leída : Display
  XY Graph : simulink/Sinks/XY Graph  xmin=-1000  xmax=1000  ymin=-1000  ymax=1000  st=-1
  Conn1 : PMIOPort  Port=1  Side=Left
  wires:
  Body Sensor/1 -> Demux/1
  Demux/2 -> Altura leída/1
  Demux/1 -> XY Graph/1, Posición X leída/1
  Demux/3 -> XY Graph/2, Posición Z leída/1
  connections:
  Conn1/RConn1 -- Body Sensor/LConn1

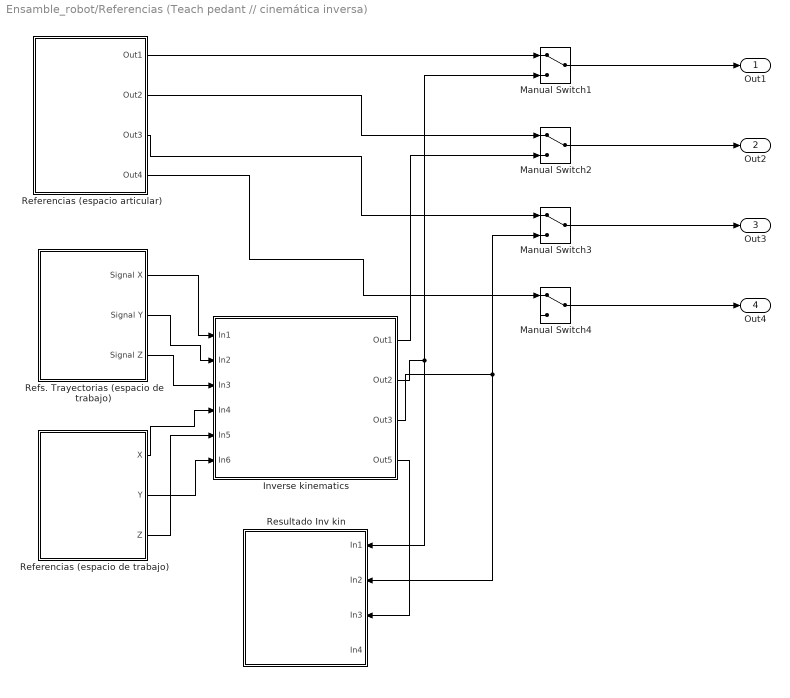
== system Ensamble_robot/Referencias (Teach pedant // cinemática inversa) ==
  Inverse kinematics : Subsystem
      mask Display: image('masks/images.jpeg');
  Manual Switch{1..4} (4 alike) : ManualSwitch
  Referencias (espacio de trabajo) : Subsystem
      mask Display: image('masks/_TEACHPD.GIF');
  Referencias (espacio articular) : Subsystem
      mask Display: image('masks/_TEACHPD.GIF');
  Refs. Trayectorias (espacio de trabajo) : Subsystem  Tag=STV Subsys  LoadFcn=sigbuilder_block('load');  StartFcn=sigbuilder_block('start');  StopFcn=sigbuilder_block('stop');  ClipboardFcn=sigbuilder_block('clipboard');  mask(Sigbuilder block){tuvar=[0:10]}
      mask help: Simulink:masks:SigbuilderBlock_MD
      mask init:
      | if ~strcmp(get_param(bdroot(gcbh),'SimulationStatus'),'stopped') tuvar = sigbuilder_block('maskInit'); end
      settings: CopyFcn=sigbuilder_block('copy');  DeleteFcn=sigbuilder_block('delete');  ModelCloseFcn=sigbuilder_block('modelClose');  PreSaveFcn=sigbuilder_block('preSave');  PauseFcn=sigbuilder_block('pause');  ContinueFcn=sigbuilder_block('continue');  NameChangeFcn=sigbuilder_block('namechange');  OpenFcn=sigbuilder_block('open',[437.6 199.2 550.4 400 ]);  CloseFcn=sigbuilder_block('close');
      mask Display: image('masks/_TEACHPD.GIF');
  Resultado Inv kin : Subsystem
      mask Display: image('masks/orion_console_2_sm.jpg');
  Out1 : Outport
  Out2 : Outport  Port=2
  Out3 : Outport  Port=3
  Out4 : Outport  Port=4
  wires:
  Inverse kinematics/2(Out2) -> Manual Switch1/2, Resultado Inv kin/1(In1)
  Inverse kinematics/3(Out3) -> Resultado Inv kin/2(In2), Manual Switch3/2
  Manual Switch2/1 -> Out2/1
  Referencias (espacio de trabajo)/3(Z) -> Inverse kinematics/5(In5)
  Refs. Trayectorias (espacio de trabajo)/3(Signal Z) -> Inverse kinematics/3(In3)
  Manual Switch3/1 -> Out3/1
  Manual Switch4/1 -> Out4/1
  Referencias (espacio de trabajo)/1(X) -> Inverse kinematics/4(In4)
  Referencias (espacio articular)/4(Out4) -> Manual Switch4/1
  Referencias (espacio articular)/1(Out1) -> Manual Switch1/1
  Referencias (espacio de trabajo)/2(Y) -> Inverse kinematics/6(In6)
  Refs. Trayectorias (espacio de trabajo)/2(Signal Y) -> Inverse kinematics/2(In2)
  Refs. Trayectorias (espacio de trabajo)/1(Signal X) -> Inverse kinematics/1(In1)
  Referencias (espacio articular)/3(Out3) -> Manual Switch3/1
  Manual Switch1/1 -> Out1/1
  Referencias (espacio articular)/2(Out2) -> Manual Switch2/1
  Inverse kinematics/4(Out5) -> Resultado Inv kin/3(In3)
  Inverse kinematics/1(Out1) -> Manual Switch2/2

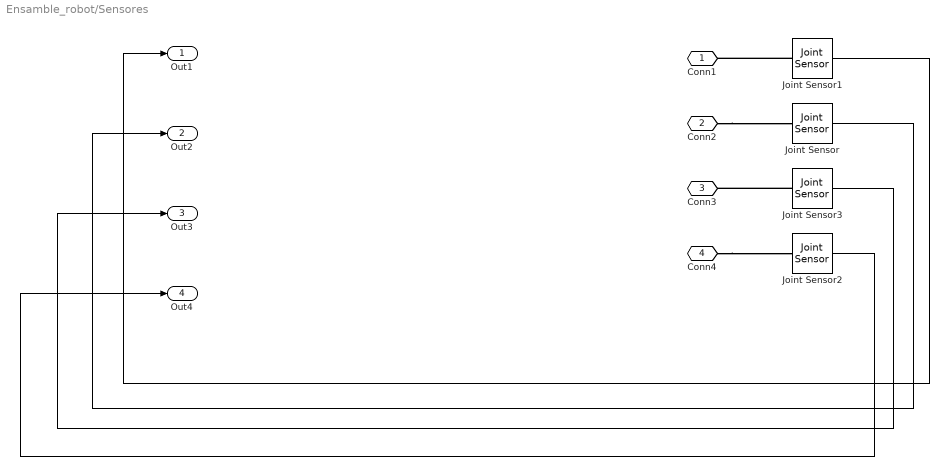
== system Ensamble_robot/Sensores ==
  Joint Sensor : mblibv1/Sensors &  Actuators/Joint Sensor  UpdateFromCAD=off  PhysicalDomain=Mechanical  PortType=blob  Muxed=on  Pose=off  Angle=on  AngleUnits=deg  ArcVelocity=off  ArcVelocityUnits=deg/s  ArcAcceleration=off  ArcAccelerationUnits=deg/s^2  CoordPosition=on  CoordPositionUnits=mm  Velocity=off  VelocityUnits=m/s  Acceleration=off  AccelerationUnits=m/s^2  Quaternion=on  QuaternionDT=off  QuaternionDDT=off  QuaternionUnits=off  OutputVector=[1]  ActiveIO=on  Width=1  DialogClass=MechanicalSensorBlock  Primitive=P1  Force=off  ForceUnits=N  Torque=off  TorqueUnits=N*m  ReferenceFrame=Absolute (World)  ReactionSensedSide=Base  ReactionReferenceFrame=Absolute (World)  ReactionForce=off  ReactionForceUnits=N  ReactionMoment=off  ReactionMomentUnits=N*m
  Joint Sensor1 : mblibv1/Sensors &  Actuators/Joint Sensor  UpdateFromCAD=off  PhysicalDomain=Mechanical  PortType=blob  Muxed=on  Pose=off  Angle=on  AngleUnits=rad  ArcVelocity=off  ArcVelocityUnits=deg/s  ArcAcceleration=off  ArcAccelerationUnits=deg/s^2  CoordPosition=on  CoordPositionUnits=mm  Velocity=off  VelocityUnits=m/s  Acceleration=off  AccelerationUnits=m/s^2  Quaternion=on  QuaternionDT=off  QuaternionDDT=off  QuaternionUnits=off  OutputVector=[1]  ActiveIO=on  Width=1  DialogClass=MechanicalSensorBlock  Primitive=R1  Force=off  ForceUnits=N  Torque=off  TorqueUnits=N*m  ReferenceFrame=Absolute (World)  ReactionSensedSide=Base  ReactionReferenceFrame=Absolute (World)  ReactionForce=off  ReactionForceUnits=N  ReactionMoment=off  ReactionMomentUnits=N*m
  Joint Sensor2 : mblibv1/Sensors &  Actuators/Joint Sensor  UpdateFromCAD=off  PhysicalDomain=Mechanical  PortType=blob  Muxed=on  Pose=off  Angle=on  AngleUnits=rad  ArcVelocity=off  ArcVelocityUnits=deg/s  ArcAcceleration=off  ArcAccelerationUnits=deg/s^2  CoordPosition=on  CoordPositionUnits=mm  Velocity=off  VelocityUnits=m/s  Acceleration=off  AccelerationUnits=m/s^2  Quaternion=on  QuaternionDT=off  QuaternionDDT=off  QuaternionUnits=off  OutputVector=[1]  ActiveIO=on  Width=1  DialogClass=MechanicalSensorBlock  Primitive=R1  Force=off  ForceUnits=N  Torque=off  TorqueUnits=N*m  ReferenceFrame=Absolute (World)  ReactionSensedSide=Base  ReactionReferenceFrame=Absolute (World)  ReactionForce=off  ReactionForceUnits=N  ReactionMoment=off  ReactionMomentUnits=N*m
  Joint Sensor3 : mblibv1/Sensors &  Actuators/Joint Sensor  UpdateFromCAD=off  PhysicalDomain=Mechanical  PortType=blob  Muxed=on  Pose=off  Angle=on  AngleUnits=rad  ArcVelocity=off  ArcVelocityUnits=deg/s  ArcAcceleration=off  ArcAccelerationUnits=deg/s^2  CoordPosition=on  CoordPositionUnits=mm  Velocity=off  VelocityUnits=m/s  Acceleration=off  AccelerationUnits=m/s^2  Quaternion=on  QuaternionDT=off  QuaternionDDT=off  QuaternionUnits=off  OutputVector=[1]  ActiveIO=on  Width=1  DialogClass=MechanicalSensorBlock  Primitive=R1  Force=off  ForceUnits=N  Torque=off  TorqueUnits=N*m  ReferenceFrame=Absolute (World)  ReactionSensedSide=Base  ReactionReferenceFrame=Absolute (World)  ReactionForce=off  ReactionForceUnits=N  ReactionMoment=off  ReactionMomentUnits=N*m
  Conn1 : PMIOPort  Port=1  Side=Left
  Conn2 : PMIOPort  Port=2  Side=Left
  Conn3 : PMIOPort  Port=3  Side=Left
  Conn4 : PMIOPort  Port=4  Side=Left
  Out1 : Outport
  Out2 : Outport  Port=2
  Out3 : Outport  Port=3
  Out4 : Outport  Port=4
  wires:
  Joint Sensor2/1 -> Out4/1
  Joint Sensor1/1 -> Out1/1
  Joint Sensor/1 -> Out2/1
  Joint Sensor3/1 -> Out3/1
  connections:
  Joint Sensor1/LConn1 -- Conn1/RConn1
  Conn2/RConn1 -- Joint Sensor/LConn1
  Joint Sensor3/LConn1 -- Conn3/RConn1
  Conn4/RConn1 -- Joint Sensor2/LConn1

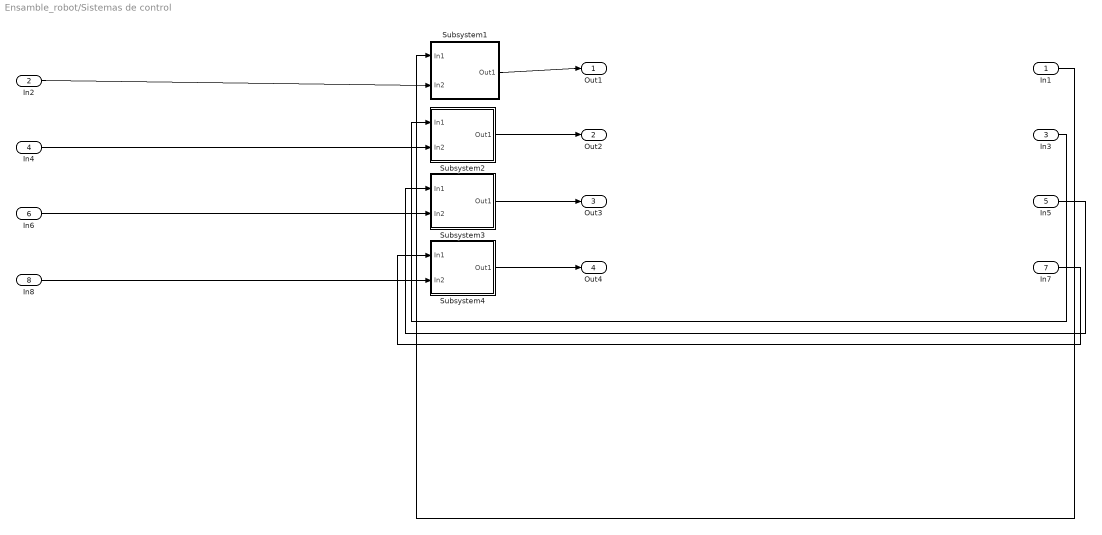
== system Ensamble_robot/Sistemas de control ==
  In1 : Inport
  In2 : Inport  Port=2
  In3 : Inport  Port=3
  In4 : Inport  Port=4
  In5 : Inport  Port=5
  In6 : Inport  Port=6
  In7 : Inport  Port=7
  In8 : Inport  Port=8
  Subsystem1 : Subsystem
  Subsystem2 : Subsystem
  Subsystem3 : Subsystem
  Subsystem4 : Subsystem
  Out1 : Outport
  Out2 : Outport  Port=2
  Out3 : Outport  Port=3
  Out4 : Outport  Port=4
  wires:
  In2/1 -> Subsystem1/2(In2)
  In8/1 -> Subsystem4/2(In2)
  In6/1 -> Subsystem3/2(In2)
  Subsystem4/1(Out1) -> Out4/1
  In7/1 -> Subsystem4/1(In1)
  Subsystem3/1(Out1) -> Out3/1
  Subsystem1/1(Out1) -> Out1/1
  In5/1 -> Subsystem3/1(In1)
  In1/1 -> Subsystem1/1(In1)
  In3/1 -> Subsystem2/1(In1)
  In4/1 -> Subsystem2/2(In2)
  Subsystem2/1(Out1) -> Out2/1

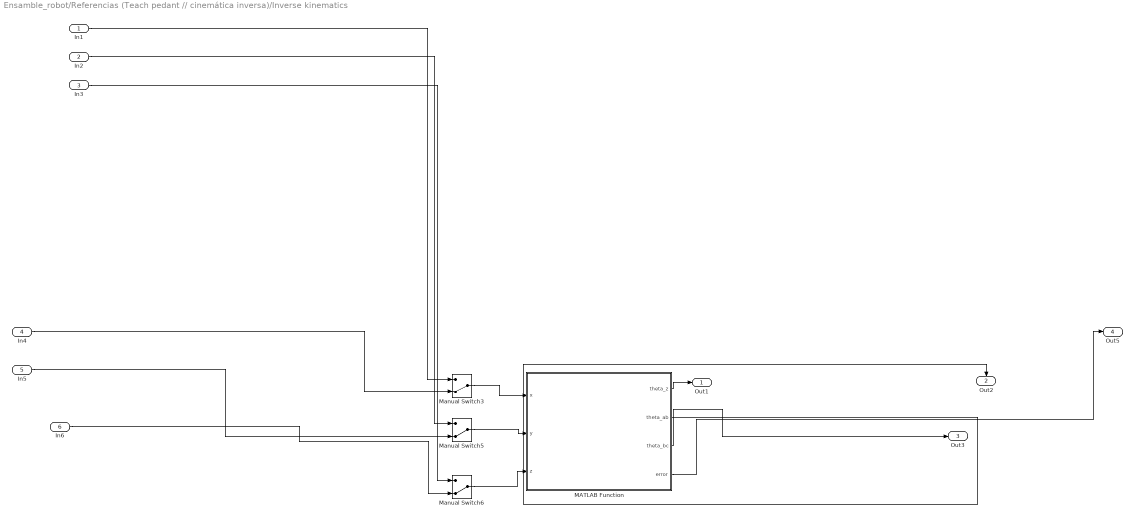
== system Ensamble_robot/Referencias (Teach pedant // cinemática inversa)/Inverse kinematics ==
  In1 : Inport
  In2 : Inport  Port=2
  In3 : Inport  Port=3
  In4 : Inport  Port=4
  In5 : Inport  Port=5
  In6 : Inport  Port=6
  MATLAB Function : MATLAB Function  TreatAsAtomicUnit=on
  Manual Switch3 : ManualSwitch  CurrentSetting=0
  Manual Switch5 : ManualSwitch  CurrentSetting=0
  Manual Switch6 : ManualSwitch  CurrentSetting=0
  Out1 : Outport
  Out2 : Outport  Port=2
  Out3 : Outport  Port=3
  Out5 : Outport  Port=4
  wires:
  MATLAB Function/4(error) -> Out5/1
  In1/1 -> Manual Switch3/1
  Manual Switch3/1 -> MATLAB Function/1(x)
  In2/1 -> Manual Switch5/1
  Manual Switch5/1 -> MATLAB Function/2(y)
  In6/1 -> Manual Switch6/2
  MATLAB Function/1(theta_z) -> Out1/1
  MATLAB Function/2(theta_ab) -> Out2/1
  MATLAB Function/3(theta_bc) -> Out3/1
  In3/1 -> Manual Switch6/1
  Manual Switch6/1 -> MATLAB Function/3(z)
  In5/1 -> Manual Switch5/2
  In4/1 -> Manual Switch3/2

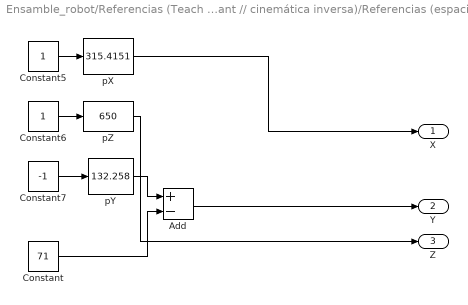
== system Ensamble_robot/Referencias (Teach pedant // cinemática inversa)/Referencias (espacio de trabajo) ==
  Add : Sum  Inputs=+-
  Constant : Constant  Value=71
  Constant5 : Constant
  Constant6 : Constant
  Constant7 : Constant  Value=-1
  pX : simulink/Math Operations/Slider Gain  low=0  gain=315.4151  high=650
  pY : simulink/Math Operations/Slider Gain  low=0  gain=132.258  high=350
  pZ : simulink/Math Operations/Slider Gain  low=-600  gain=650  high=650
  X : Outport
  Y : Outport  Port=2
  Z : Outport  Port=3
  wires:
  Add/1 -> Y/1
  pX/1 -> X/1
  pZ/1 -> Z/1
  Constant5/1 -> pX/1
  pY/1 -> Add/1
  Constant7/1 -> pY/1
  Constant6/1 -> pZ/1
  Constant/1 -> Add/2

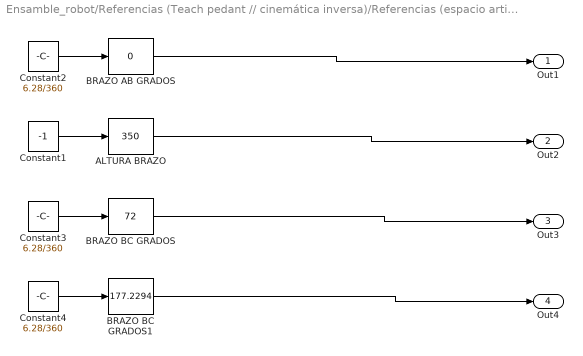
== system Ensamble_robot/Referencias (Teach pedant // cinemática inversa)/Referencias (espacio articular) ==
  ALTURA BRAZO : simulink/Math Operations/Slider Gain  low=0  gain=350  high=350
  BRAZO AB GRADOS : simulink/Math Operations/Slider Gain  low=0  gain=0  high=180
  BRAZO BC GRADOS : simulink/Math Operations/Slider Gain  low=0  gain=72  high=180
  BRAZO BC GRADOS1 : simulink/Math Operations/Slider Gain  low=0  gain=177.2294  high=180
  Constant1 : Constant  Value=-1
  Constant2 : Constant  Value=6.28/360
  Constant3 : Constant  Value=6.28/360
  Constant4 : Constant  Value=6.28/360
  Out1 : Outport
  Out2 : Outport  Port=2
  Out3 : Outport  Port=3
  Out4 : Outport  Port=4
  wires:
  Constant4/1 -> BRAZO BC GRADOS1/1
  ALTURA BRAZO/1 -> Out2/1
  Constant1/1 -> ALTURA BRAZO/1
  BRAZO AB GRADOS/1 -> Out1/1
  Constant2/1 -> BRAZO AB GRADOS/1
  BRAZO BC GRADOS1/1 -> Out4/1
  BRAZO BC GRADOS/1 -> Out3/1
  Constant3/1 -> BRAZO BC GRADOS/1

== system Ensamble_robot/Referencias (Teach pedant // cinemática inversa)/Refs. Trayectorias (espacio de trabajo) ==
  Demux : Demux  Tag=STV Demux  Outputs=3
  FromWs : FromWorkspace  Tag=STV FromWs  VariableName=tuvar  SampleTime=0
      SigBuilderData=|
      | common.afterFinalStr = 'Extrapolate'
      | common.sampleTime = 0
      | dataSet.timeRange = [0 10]
      | dataSet.name = 'Group 1'
      | sbobj.Groups.Name = 'Group 1'
      | sbobj.Groups.Signals(1).Name = 'Signal X'
      | sbobj.Groups.Signals(1).XData = [0 6 6 10]
      | sbobj.Groups.Signals(1).YData = [-0.085 1 0 0]
      | sbobj.Groups.Signals(2).Name = 'Signal Y'
      | sbobj.Groups.Signals(2).XData = [0 1 2 3 4 5 6 7 8 9 10]
      | sbobj.Groups.Signals(2).YData = [1 1 1 1 1 1 1 1 1 1 1]
      | sbobj.Groups.Signals(3).Name = 'Signal Z'
      | sbobj.Groups.Signals(3).XData = [0 4 4 6 6 10]
      | sbobj.Groups.Signals(3).YData = [0 0 1 1 0 0]
  Signal X : Outport  Tag=STV Outport
  Signal Y : Outport  Tag=STV Outport  Port=2
  Signal Z : Outport  Tag=STV Outport  Port=3
  wires:
  Demux/1 -> Signal X/1
  FromWs/1 -> Demux/1
  Demux/2 -> Signal Y/1
  Demux/3 -> Signal Z/1

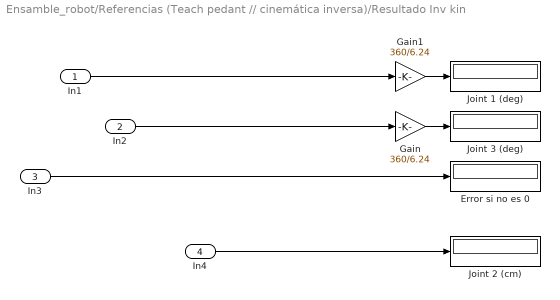
== system Ensamble_robot/Referencias (Teach pedant // cinemática inversa)/Resultado Inv kin ==
  In1 : Inport
  In2 : Inport  Port=2
  In3 : Inport  Port=3
  In4 : Inport  Port=4
  "Error si no es 0 " : Display
  Gain : Gain  Gain=360/6.24
  Gain1 : Gain  Gain=360/6.24
  Joint 1 (deg) : Display
  Joint 2 (cm) : Display
  "Joint 3 (deg) " : Display
  wires:
  In4/1 -> Joint 2 (cm)/1
  In1/1 -> Gain1/1
  In2/1 -> Gain/1
  Gain1/1 -> Joint 1 (deg)/1
  Gain/1 -> "Joint 3 (deg) "/1
  In3/1 -> "Error si no es 0 "/1

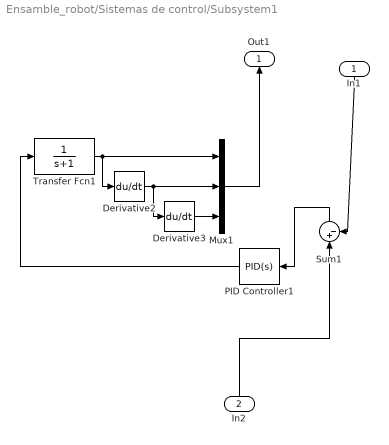
== system Ensamble_robot/Sistemas de control/Subsystem1 ==
  In1 : Inport
  In2 : Inport  Port=2
  Derivative2 : Derivative
  Derivative3 : Derivative
  Mux1 : Mux  Inputs=3
  PID Controller1 : simulink/Continuous/PID Controller  Controller=PID  TimeDomain=Continuous-time  SampleTime=-1  IntegratorMethod=Forward Euler  FilterMethod=Forward Euler  Form=Parallel  UseFilter=on  ControllerParametersSource=internal  P=1  I=1  D=0  N=100  InitialConditionSource=internal  InitialConditionForIntegrator=0  InitialConditionForFilter=0  ExternalReset=none  LimitOutput=on  UpperSaturationLimit=500  LowerSaturationLimit=-500  LinearizeAsGain=on  AntiWindupMode=none  Kb=1  TrackingMode=off  Kt=1  PParamMin=[]  PParamMax=[]  IParamMin=[]  IParamMax=[]  DParamMin=[]  DParamMax=[]  NParamMin=[]  NParamMax=[]  KbParamMin=[]  KbParamMax=[]  KtParamMin=[]  KtParamMax=[]  POutMin=[]  POutMax=[]  IOutMin=[]  IOutMax=[]  DOutMin=[]  DOutMax=[]  NOutMin=[]  NOutMax=[]  KbOutMin=[]  KbOutMax=[]  KtOutMin=[]  KtOutMax=[]  IntegratorOutMin=[]  IntegratorOutMax=[]  FilterOutMin=[]  FilterOutMax=[]  SumOutMin=[]  SumOutMax=[]  SumI1OutMin=[]  SumI1OutMax=[]  SumI2OutMin=[]  SumI2OutMax=[]  SumI3OutMin=[]  SumI3OutMax=[]  SumDOutMin=[]  SumDOutMax=[]  SaturationOutMin=[]  SaturationOutMax=[]  IntegratorContinuousStateAttributes=''  IntegratorStateMustResolveToSignalObject=off  IntegratorRTWStateStorageClass=Auto  FilterContinuousStateAttributes=''  FilterStateMustResolveToSignalObject=off  FilterRTWStateStorageClass=Auto  DifferentiatorICPrevScaledInput=0  DifferentiatorOutMin=[]  DifferentiatorOutMax=[]
  Sum1 : Sum  Inputs=|+-
  Transfer Fcn1 : TransferFcn  Denominator=[1 1]
  Out1 : Outport
  wires:
  Derivative3/1 -> Mux1/3
  PID Controller1/1 -> Transfer Fcn1/1
  Mux1/1 -> Out1/1
  In1/1 -> Sum1/2
  Sum1/1 -> PID Controller1/1
  Derivative2/1 -> Derivative3/1, Mux1/2
  Transfer Fcn1/1 -> Derivative2/1, Mux1/1
  In2/1 -> Sum1/1

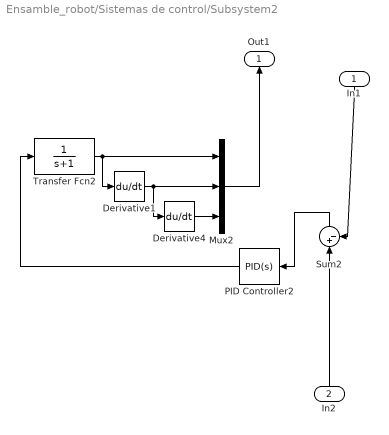
== system Ensamble_robot/Sistemas de control/Subsystem2 ==
  In1 : Inport
  In2 : Inport  Port=2
  Derivative1 : Derivative
  Derivative4 : Derivative
  Mux2 : Mux  Inputs=3
  PID Controller2 : simulink/Continuous/PID Controller  Controller=PID  TimeDomain=Continuous-time  SampleTime=-1  IntegratorMethod=Forward Euler  FilterMethod=Forward Euler  Form=Parallel  UseFilter=on  ControllerParametersSource=internal  P=1  I=1  D=0  N=100  InitialConditionSource=internal  InitialConditionForIntegrator=0  InitialConditionForFilter=0  ExternalReset=none  LimitOutput=on  UpperSaturationLimit=500  LowerSaturationLimit=-500  LinearizeAsGain=on  AntiWindupMode=none  Kb=1  TrackingMode=off  Kt=1  PParamMin=[]  PParamMax=[]  IParamMin=[]  IParamMax=[]  DParamMin=[]  DParamMax=[]  NParamMin=[]  NParamMax=[]  KbParamMin=[]  KbParamMax=[]  KtParamMin=[]  KtParamMax=[]  POutMin=[]  POutMax=[]  IOutMin=[]  IOutMax=[]  DOutMin=[]  DOutMax=[]  NOutMin=[]  NOutMax=[]  KbOutMin=[]  KbOutMax=[]  KtOutMin=[]  KtOutMax=[]  IntegratorOutMin=[]  IntegratorOutMax=[]  FilterOutMin=[]  FilterOutMax=[]  SumOutMin=[]  SumOutMax=[]  SumI1OutMin=[]  SumI1OutMax=[]  SumI2OutMin=[]  SumI2OutMax=[]  SumI3OutMin=[]  SumI3OutMax=[]  SumDOutMin=[]  SumDOutMax=[]  SaturationOutMin=[]  SaturationOutMax=[]  IntegratorContinuousStateAttributes=''  IntegratorStateMustResolveToSignalObject=off  IntegratorRTWStateStorageClass=Auto  FilterContinuousStateAttributes=''  FilterStateMustResolveToSignalObject=off  FilterRTWStateStorageClass=Auto  DifferentiatorICPrevScaledInput=0  DifferentiatorOutMin=[]  DifferentiatorOutMax=[]
  Sum2 : Sum  Inputs=|+-
  Transfer Fcn2 : TransferFcn  Denominator=[1 1]
  Out1 : Outport
  wires:
  Transfer Fcn2/1 -> Derivative1/1, Mux2/1
  Derivative1/1 -> Derivative4/1, Mux2/2
  Sum2/1 -> PID Controller2/1
  Derivative4/1 -> Mux2/3
  PID Controller2/1 -> Transfer Fcn2/1
  Mux2/1 -> Out1/1
  In2/1 -> Sum2/1
  In1/1 -> Sum2/2

== system Ensamble_robot/Sistemas de control/Subsystem3 ==
  In1 : Inport
  In2 : Inport  Port=2
  Derivative5 : Derivative
  Derivative6 : Derivative
  Mux3 : Mux  Inputs=3
  PID Controller3 : simulink/Continuous/PID Controller  Controller=PID  TimeDomain=Continuous-time  SampleTime=-1  IntegratorMethod=Forward Euler  FilterMethod=Forward Euler  Form=Parallel  UseFilter=on  ControllerParametersSource=internal  P=1  I=1  D=0  N=100  InitialConditionSource=internal  InitialConditionForIntegrator=0  InitialConditionForFilter=0  ExternalReset=none  LimitOutput=on  UpperSaturationLimit=500  LowerSaturationLimit=-500  LinearizeAsGain=on  AntiWindupMode=none  Kb=1  TrackingMode=off  Kt=1  PParamMin=[]  PParamMax=[]  IParamMin=[]  IParamMax=[]  DParamMin=[]  DParamMax=[]  NParamMin=[]  NParamMax=[]  KbParamMin=[]  KbParamMax=[]  KtParamMin=[]  KtParamMax=[]  POutMin=[]  POutMax=[]  IOutMin=[]  IOutMax=[]  DOutMin=[]  DOutMax=[]  NOutMin=[]  NOutMax=[]  KbOutMin=[]  KbOutMax=[]  KtOutMin=[]  KtOutMax=[]  IntegratorOutMin=[]  IntegratorOutMax=[]  FilterOutMin=[]  FilterOutMax=[]  SumOutMin=[]  SumOutMax=[]  SumI1OutMin=[]  SumI1OutMax=[]  SumI2OutMin=[]  SumI2OutMax=[]  SumI3OutMin=[]  SumI3OutMax=[]  SumDOutMin=[]  SumDOutMax=[]  SaturationOutMin=[]  SaturationOutMax=[]  IntegratorContinuousStateAttributes=''  IntegratorStateMustResolveToSignalObject=off  IntegratorRTWStateStorageClass=Auto  FilterContinuousStateAttributes=''  FilterStateMustResolveToSignalObject=off  FilterRTWStateStorageClass=Auto  DifferentiatorICPrevScaledInput=0  DifferentiatorOutMin=[]  DifferentiatorOutMax=[]
  Sum3 : Sum  Inputs=|+-
  Transfer Fcn3 : TransferFcn  Denominator=[1 1]
  Out1 : Outport
  wires:
  Mux3/1 -> Out1/1
  In1/1 -> Sum3/2
  Derivative6/1 -> Mux3/3
  In2/1 -> Sum3/1
  Sum3/1 -> PID Controller3/1
  PID Controller3/1 -> Transfer Fcn3/1
  Derivative5/1 -> Derivative6/1, Mux3/2
  Transfer Fcn3/1 -> Derivative5/1, Mux3/1

== system Ensamble_robot/Sistemas de control/Subsystem4 ==
  In1 : Inport
  In2 : Inport  Port=2
  Derivative7 : Derivative
  Derivative8 : Derivative
  Mux4 : Mux  Inputs=3
  PID Controller4 : simulink/Continuous/PID Controller  Controller=PID  TimeDomain=Continuous-time  SampleTime=-1  IntegratorMethod=Forward Euler  FilterMethod=Forward Euler  Form=Parallel  UseFilter=on  ControllerParametersSource=internal  P=1  I=1  D=0  N=100  InitialConditionSource=internal  InitialConditionForIntegrator=0  InitialConditionForFilter=0  ExternalReset=none  LimitOutput=on  UpperSaturationLimit=500  LowerSaturationLimit=-500  LinearizeAsGain=on  AntiWindupMode=none  Kb=1  TrackingMode=off  Kt=1  PParamMin=[]  PParamMax=[]  IParamMin=[]  IParamMax=[]  DParamMin=[]  DParamMax=[]  NParamMin=[]  NParamMax=[]  KbParamMin=[]  KbParamMax=[]  KtParamMin=[]  KtParamMax=[]  POutMin=[]  POutMax=[]  IOutMin=[]  IOutMax=[]  DOutMin=[]  DOutMax=[]  NOutMin=[]  NOutMax=[]  KbOutMin=[]  KbOutMax=[]  KtOutMin=[]  KtOutMax=[]  IntegratorOutMin=[]  IntegratorOutMax=[]  FilterOutMin=[]  FilterOutMax=[]  SumOutMin=[]  SumOutMax=[]  SumI1OutMin=[]  SumI1OutMax=[]  SumI2OutMin=[]  SumI2OutMax=[]  SumI3OutMin=[]  SumI3OutMax=[]  SumDOutMin=[]  SumDOutMax=[]  SaturationOutMin=[]  SaturationOutMax=[]  IntegratorContinuousStateAttributes=''  IntegratorStateMustResolveToSignalObject=off  IntegratorRTWStateStorageClass=Auto  FilterContinuousStateAttributes=''  FilterStateMustResolveToSignalObject=off  FilterRTWStateStorageClass=Auto  DifferentiatorICPrevScaledInput=0  DifferentiatorOutMin=[]  DifferentiatorOutMax=[]
  Sum4 : Sum  Inputs=|+-
  Transfer Fcn4 : TransferFcn  Denominator=[1 1]
  Out1 : Outport
  wires:
  Derivative8/1 -> Mux4/3
  Mux4/1 -> Out1/1
  In2/1 -> Sum4/1
  Transfer Fcn4/1 -> Derivative7/1, Mux4/1
  Sum4/1 -> PID Controller4/1
  In1/1 -> Sum4/2
  PID Controller4/1 -> Transfer Fcn4/1
  Derivative7/1 -> Derivative8/1, Mux4/2

== matlab function Ensamble_robot/Referencias (Teach pedant // cinemática inversa)/Inverse kinematics/MATLAB Function ==
  data: x input; theta_z output; y input; z input; theta_ab output; theta_bc output; error output
function [theta_z,theta_ab,theta_bc,error]=fcn(x,y,z)
%function [theta_z,theta_ab,theta_bc,error,xb,yb,zb]=fcn(x,y,z)
%Función para resolver el problema de la posición inverso para un modo de
%ensamblaje del robot angular
%
%Entradas
%x (coordenada X del extremo del robot)
%y (coordenada Y del extremo del robot)
%z (coordenada Z del extremo del robot)
%
%Salidas
%theta_z (ángulo de la proyección de ABC respecto al semieje X sobre el plano XOY)
%theta_ab (ángulo del segmento AB respecto al semieje U)
%theta_bc (ángulo del segmento BC respecto al semieje U)
%error (Error de montaje)
%xb (coordenada X de la articulación B)
%yb (coordenada Y de la articulación B)
%zb (coordenada Z de la articulación B)
%
%                                   CODIGO
%Definir las variables globales
 %global loa lab lbc
    loa=596;
    lab=450;
    lbc=200;
    
    
%Calcular la distancia OC proyectada en U
    loc=sqrt(x^2+y^2);
    
%Calcular el ángulo theta_Z
    theta_z=atan2(y,x);
    
%Definir las coordenadas de A y B en el plano UOZ
    xa=0;
    ya=0;
    xc=x;
    yc=y;
    %za=loa;
    
   % uc=loc;
   % zc=z;
    
%Calcular la posición de B con el modo de ensamblaje 1
    [xb,yb,error]=RRR(xa,ya,xc,yc,lab,lbc,1);
    
%Calcular los ángulos theta_ab y theta_bc
    theta_ab=atan2(yb,xb);
    theta_bc=atan2(yc-yb,xc-xb);

%Calcular la posición global de B
%     xb=lab*cos(theta_ab)*cos(theta_z);
%     yb=lab*cos(theta_ab)*sin(theta_z);
    
    %zb=loa+lab*sin(theta_ab);
    zb=z;
